simulink model "UNO_PWMout_task"  (Simulink 3.00)
settings: Solver=ode45  SolverMode=SingleTasking  StartTime=0.0  StopTime=10.0  RelTol=1e-3
libraries: analoglib x5, mathlib x5, REXduino_library x1, genlib x1
settings Model: Creator=Jarda  LastModifiedBy=XPMUser

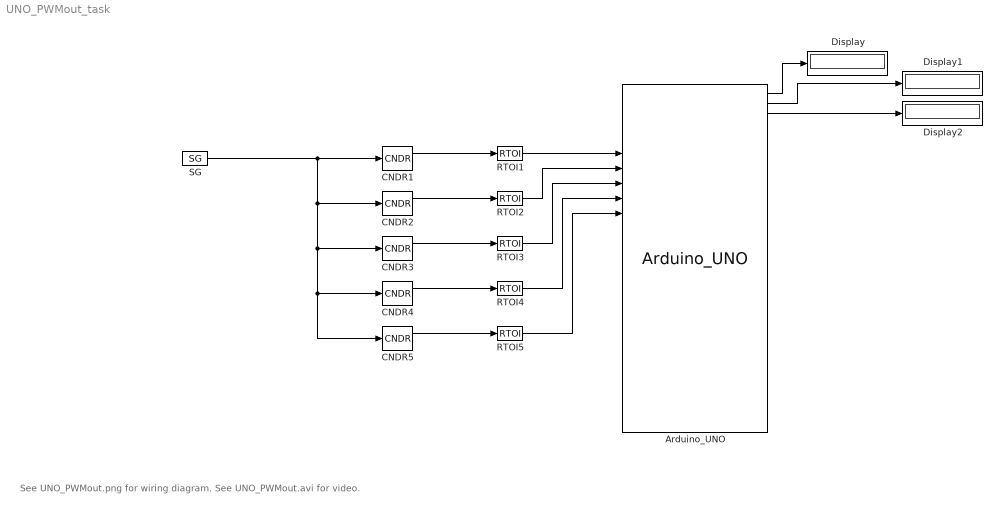
== system UNO_PWMout_task ==
  note: See UNO_PWMout.png for wiring diagram.
      |
      | See UNO_PWMout.avi for video.
  Arduino_UNO : REXduino_library/Arduino_UNO  comPort=/dev/ttyACM0  pinmode2=1: Not connected  pinmode3=1: Not connected  pinmode4=1: Not connected  pinmode5=5: PWM (analog output)  pinmode6=5: PWM (analog output)  pinmode9=5: PWM (analog output)  pinmode10=5: PWM (analog output)  pinmode11=5: PWM (analog output)  pinmodeA0=1: Not connected  pinmodeA1=1: Not connected  pinmodeA2=1: Not connected  pinmodeA3=1: Not connected  pinmodeA4=1: Not connected  pinmodeA5=1: Not connected
  CNDR1 : analoglib/CNDR  n=4  SATF=on  up=[-1 -0.6 0.6 1]  yp=[255 0 0 255]
  CNDR2 : analoglib/CNDR  n=3  SATF=on  up=[-1 -0.6 -0.2]  yp=[0 255 0]
  CNDR3 : analoglib/CNDR  n=3  SATF=on  up=[-0.6 -0.2 0.2]  yp=[0 255 0]
  CNDR4 : analoglib/CNDR  n=3  SATF=on  up=[-0.2 0.2 0.6]  yp=[0 255 0]
  CNDR5 : analoglib/CNDR  n=3  SATF=on  up=[0.2 0.6 1]  yp=[0 255 0]
  Display : Display
      settings: Format=Best fit
  Display1 : Display
      settings: Format=Best fit
  Display2 : Display
      settings: Format=Best fit
  RTOI{1..5} (5 alike) : mathlib/RTOI
  SG : genlib/SG  isig=3: SAWTOOTH  amp=1  freq=2  phase=0  ifrunit=1: Hz  iphunit=1: degrees  offset=0
  wires:
  Arduino_UNO/1 -> Display/1
  Arduino_UNO/2 -> Display1/1
  Arduino_UNO/3 -> Display2/1
  CNDR1/1 -> RTOI1/1
  CNDR2/1 -> RTOI2/1
  CNDR3/1 -> RTOI3/1
  CNDR4/1 -> RTOI4/1
  CNDR5/1 -> RTOI5/1
  RTOI1/1 -> Arduino_UNO/4
  RTOI2/1 -> Arduino_UNO/5
  RTOI3/1 -> Arduino_UNO/6
  RTOI4/1 -> Arduino_UNO/7
  RTOI5/1 -> Arduino_UNO/8
  SG/1 -> CNDR1/1, CNDR2/1, CNDR3/1, CNDR4/1, CNDR5/1
